simulink model "simulink_old_control_code"  (R2022b)
settings: Solver=FixedStepAuto  StartTime=0.0  StopTime=inf  FixedStep=0.0002  RelTol=1e-3
values from neighbouring files (symbols this model uses):
  bias_heave1 = 0    [setup_DAQ_simulink_temp.m]
  freq = 0.65    [setup_DAQ_simulink_temp.m]
  heave1 = hstar1*chord    [setup_DAQ_simulink_temp.m]
  phase = -60    [setup_DAQ_simulink_temp.m]
  phi = -90    [setup_DAQ_simulink_temp.m]
  srate = 1000    [setup_DAQ_simulink_temp.m]
  T = 1/srate    (= 0.001)    [setup_DAQ_simulink_temp.m]
undefined symbols (not defined in the file or in its folder): bias_forces, National_Instruments, PCIe, Wallace_cal_transpose
libraries: sldrtlib x13
settings Model: SimulationMode=external  ExtModeTrigPort=2  ExtModeTrigDuration=6000000  ExtModeTrigDurationFloating=inf  ExtModeTrigLevel=0.500000  Creator=xhe61  LastModifiedBy=ehandyca
settings DataIOCC: ReturnWorkspaceOutputs=off
settings HardwareCC: ProdBitPerLong=64  ProdHWDeviceType=Intel->x86-64 (Linux 64)
settings ModelReferenceCC: EnableRefExpFcnMdlSchedulingChecks=on
settings RTWCC: Description=Simulink Desktop Real-Time  SystemTargetFile=sldrt.tlc  TemplateMakefile=sldrt.tmf  RTWCompilerOptimization=on
settings CodeAppCC: MaxIdLength=95
settings SimulinkDesktopRealTimeCC: TargetLibSuffix=_sldrt.a  TargetPreCompLibLocation=C:\Program Files\MATLAB\R2022b\toolbox\sldrt\lib\win64

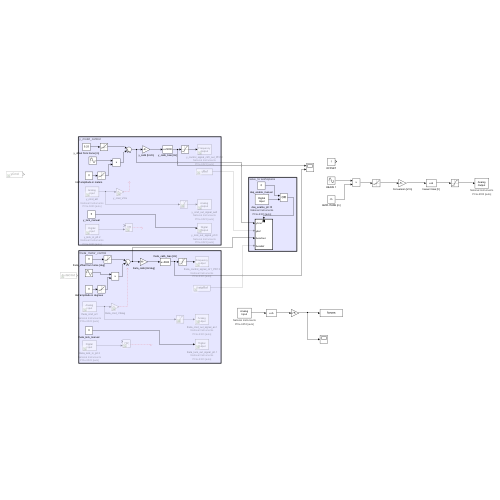
[thumbnail: Simulink's stored preview of the top-level diagram]
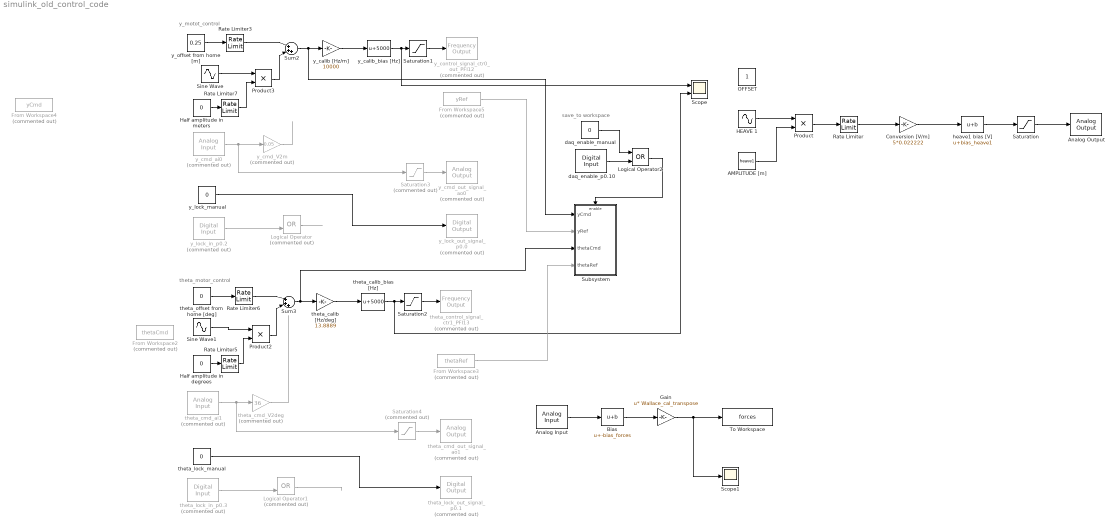
== system simulink_old_control_code ==
  note: save_to workspace
  note: theta_motor_control
  note: y_motot_control
  AMPLITUDE [m] : Constant  Value=heave1
  Analog Input : sldrtlib/Analog Input  SampleTime=T  MaxMissedTicks=10  ShowMissedTicks=off  YieldWhenWaiting=off  DrvName=National_Instruments/PCIe-6353  DrvAddress=4294967295  DrvOptions=[1 0 0 2 2 2 2]  Channels=[1:6]  RangeMode=1  VoltRange=1  DataType=1
      settings: AttributesFormatString=National Instruments\nPCIe-6353 [auto]
  Analog Output : sldrtlib/Analog Output  SampleTime=srate  MaxMissedTicks=10  ShowMissedTicks=off  YieldWhenWaiting=off  DrvName=National_Instruments/PCIe-6353  DrvAddress=4294967295  DrvOptions=[1 0 0 2 2 2 2]  Channels=1  RangeMode=1  VoltRange=1  InitialValue=[]  FinalValue=[]
      settings: AttributesFormatString=National Instruments\nPCIe-6353 [auto]
  Bias : Bias  Bias=-bias_forces  SaturateOnIntegerOverflow=off
  Conversion [V/m] : Gain  Gain=5*0.022222
  From Workspace2 : FromWorkspace  Commented=on  VariableName=thetaCmd  SampleTime=0.001  Interpolate=off  OutputAfterFinalValue=Cyclic repetition
  From Workspace3 : FromWorkspace  Commented=on  VariableName=thetaRef  SampleTime=0.001  Interpolate=off  OutputAfterFinalValue=Cyclic repetition
  From Workspace4 : FromWorkspace  Commented=on  VariableName=yCmd  SampleTime=0.001  Interpolate=off  OutputAfterFinalValue=Cyclic repetition
  From Workspace5 : FromWorkspace  Commented=on  VariableName=yRef  SampleTime=0.001  Interpolate=off  OutputAfterFinalValue=Cyclic repetition
  Gain : Gain  Gain=Wallace_cal_transpose  Multiplication=Matrix(u*K)
  HEAVE 1 : Sin  Frequency=freq  Phase=phase + phi  SampleTime=0
  Half amplitude in degrees : Constant  Value=0
  Half amplitude in meters : Constant  Value=0
  Logical Operator : Logic  Commented=on  Operator=OR  AllPortsSameDT=off  OutDataTypeStr=boolean
  Logical Operator1 : Logic  Commented=on  Operator=OR  AllPortsSameDT=off  OutDataTypeStr=boolean
  Logical Operator2 : Logic  Operator=OR  AllPortsSameDT=off  OutDataTypeStr=boolean
  OFFSET : Constant
  Product : Product
  Product2 : Product
  Product3 : Product
  Rate Limiter : RateLimiter  SampleTimeMode=inherited
  Rate Limiter3 : RateLimiter  RisingSlewLimit=0.04  FallingSlewLimit=-0.04  SampleTimeMode=inherited
  Rate Limiter5 : RateLimiter  RisingSlewLimit=10  FallingSlewLimit=-10  SampleTimeMode=inherited
  Rate Limiter6 : RateLimiter  RisingSlewLimit=15  FallingSlewLimit=-15  SampleTimeMode=inherited
  Rate Limiter7 : RateLimiter  RisingSlewLimit=0.01  FallingSlewLimit=-0.01  SampleTimeMode=inherited
  Saturation : Saturate  UpperLimit=10  LowerLimit=-10
  Saturation1 : Saturate  UpperLimit=10000  LowerLimit=5000
  Saturation2 : Saturate  UpperLimit=9200  LowerLimit=5000
  Saturation3 : Saturate  Commented=on  UpperLimit=10  LowerLimit=-10
  Saturation4 : Saturate  Commented=on  UpperLimit=10  LowerLimit=-10
  Scope : Scope  NumInputPorts=2
  Scope1 : Scope
  Sine Wave : Sin  Frequency=2*pi*0.65  SampleTime=0
  Sine Wave1 : Sin  Frequency=2*pi*0.65  Phase=-pi/2  SampleTime=0
  Subsystem : Subsystem
  Sum2 : Sum  Inputs=|+++
  Sum3 : Sum  Inputs=|+++
  To Workspace : ToWorkspace  VariableName=forces  SampleTime=-1
      settings: MaxDataPoints=20000  Save2DSignal=2-D array (concatenate along first dimension)
  daq_enable_manual : Constant  Value=0  OutDataTypeStr=boolean
  daq_enable_p0.10 : sldrtlib/Digital Input  SampleTime=0.001  MaxMissedTicks=10  ShowMissedTicks=off  YieldWhenWaiting=on  DrvName=National_Instruments/PCIe-6323  DrvAddress=4294967295  DrvOptions=[0 3 0 3 3 3 3]  Channels=11  BitMode=1  DataType=9
      settings: AttributesFormatString=National Instruments\nPCIe-6323 [auto]
  heave1 bias [V] : Bias  Bias=bias_heave1  SaturateOnIntegerOverflow=off
  theta_calib [Hz/deg] : Gain  Gain=13.8889
  theta_calib_bias [Hz] : Bias  Bias=5000  SaturateOnIntegerOverflow=off
  theta_cmd_V2deg : Gain  Commented=on  Gain=36
  theta_cmd_ai1 : sldrtlib/Analog Input  Commented=on  SampleTime=0.001  MaxMissedTicks=10  ShowMissedTicks=off  YieldWhenWaiting=off  DrvName=National_Instruments/PCIe-6323  DrvAddress=4294967295  DrvOptions=[0 3 61440 3 3 3 3]  Channels=2  RangeMode=1  VoltRange=1  DataType=1
      settings: AttributesFormatString=National Instruments\nPCIe-6323 [auto]
  theta_cmd_out_signal_ao1 : sldrtlib/Analog Output  Commented=on  SampleTime=0.001  MaxMissedTicks=10  ShowMissedTicks=off  YieldWhenWaiting=off  DrvName=National_Instruments/PCIe-6323  DrvAddress=4294967295  DrvOptions=[0 3 61440 3 3 3 3]  Channels=2  RangeMode=1  VoltRange=1  InitialValue=[]  FinalValue=[]
      settings: AttributesFormatString=National Instruments\nPCIe-6323 [auto]
  theta_control_signal_ctr1_PFI13 : sldrtlib/Frequency Output  Commented=on  SampleTime=T  MaxMissedTicks=10  ShowMissedTicks=off  YieldWhenWaiting=off  DrvName=National_Instruments/PCIe-6323  DrvAddress=4294967295  DrvOptions=[0 3 0 3 3 3 3]  Channels=2  FrequencySource=2  Frequency=[]  FrequencyFinalValue=[]  DutySource=1  Duty=0.5  DutyFinalValue=[]
      settings: AttributesFormatString=National Instruments\nPCIe-6323 [auto]
  theta_lock_in_p0.3 : sldrtlib/Digital Input  Commented=on  SampleTime=0.001  MaxMissedTicks=10  ShowMissedTicks=off  YieldWhenWaiting=on  DrvName=National_Instruments/PCIe-6323  DrvAddress=4294967295  DrvOptions=[0 3 61440 3 3 3 3]  Channels=4  BitMode=1  DataType=9
      settings: AttributesFormatString=National Instruments\nPCIe-6323 [auto]
  theta_lock_manual : Constant  Value=0  OutDataTypeStr=boolean
  theta_lock_out_signal_p0.1 : sldrtlib/Digital Output  Commented=on  SampleTime=T  MaxMissedTicks=10  ShowMissedTicks=off  YieldWhenWaiting=off  DrvName=National_Instruments/PCIe-6323  DrvAddress=4294967295  DrvOptions=[0 3 0 3 3 3 3]  Channels=2  BitMode=1  InitialValue=[]  FinalValue=[]
      settings: AttributesFormatString=National Instruments\nPCIe-6323 [auto]
  theta_offset from home [deg] : Constant  Value=0
  y_calib [Hz/m] : Gain  Gain=10000
  y_calib_bias [Hz] : Bias  Bias=5000  SaturateOnIntegerOverflow=off
  y_cmd_V2m : Gain  Commented=on  Gain=0.05
  y_cmd_ai0 : sldrtlib/Analog Input  Commented=on  SampleTime=0.001  MaxMissedTicks=10  ShowMissedTicks=off  YieldWhenWaiting=off  DrvName=National_Instruments/PCIe-6323  DrvAddress=4294967295  DrvOptions=[0 3 61440 3 3 3 3]  Channels=1  RangeMode=1  VoltRange=1  DataType=1
      settings: AttributesFormatString=National Instruments\nPCIe-6323 [auto]
  y_cmd_out_signal_ao0 : sldrtlib/Analog Output  Commented=on  SampleTime=0.001  MaxMissedTicks=10  ShowMissedTicks=off  YieldWhenWaiting=off  DrvName=National_Instruments/PCIe-6323  DrvAddress=4294967295  DrvOptions=[0 3 61440 3 3 3 3]  Channels=1  RangeMode=1  VoltRange=1  InitialValue=[]  FinalValue=[]
      settings: AttributesFormatString=National Instruments\nPCIe-6323 [auto]
  y_control_signal_ctr0_out_PFI12 : sldrtlib/Frequency Output  Commented=on  SampleTime=T  MaxMissedTicks=10  ShowMissedTicks=off  YieldWhenWaiting=off  DrvName=National_Instruments/PCIe-6323  DrvAddress=4294967295  DrvOptions=[0 3 0 3 3 3 3]  Channels=1  FrequencySource=2  Frequency=[]  FrequencyFinalValue=[]  DutySource=1  Duty=0.5  DutyFinalValue=[]
      settings: AttributesFormatString=National Instruments\nPCIe-6323 [auto]
  y_lock_in_p0.2 : sldrtlib/Digital Input  Commented=on  SampleTime=0.001  MaxMissedTicks=10  ShowMissedTicks=off  YieldWhenWaiting=on  DrvName=National_Instruments/PCIe-6323  DrvAddress=4294967295  DrvOptions=[0 3 61440 3 3 3 3]  Channels=3  BitMode=1  DataType=9
      settings: AttributesFormatString=National Instruments\nPCIe-6323 [auto]
  y_lock_manual : Constant  Value=0  OutDataTypeStr=boolean
  y_lock_out_signal_p0.0 : sldrtlib/Digital Output  Commented=on  SampleTime=T  MaxMissedTicks=10  ShowMissedTicks=off  YieldWhenWaiting=off  DrvName=National_Instruments/PCIe-6323  DrvAddress=4294967295  DrvOptions=[0 3 0 3 3 3 3]  Channels=1  BitMode=1  InitialValue=[]  FinalValue=[]
      settings: AttributesFormatString=National Instruments\nPCIe-6323 [auto]
  y_offset from home [m] : Constant  Value=0.25
  wires:
  y_lock_manual/1 -> y_lock_out_signal_p0.0/1
  theta_lock_in_p0.3/1 -> Logical Operator1/2
  theta_lock_manual/1 -> theta_lock_out_signal_p0.1/1
  y_cmd_ai0/1 -> Saturation3/1, y_cmd_V2m/1
  Logical Operator/1 -> ?
  Saturation4/1 -> theta_cmd_out_signal_ao1/1
  theta_cmd_ai1/1 -> theta_cmd_V2deg/1, Saturation4/1
  theta_cmd_V2deg/1 -> ?
  y_offset from home [m]/1 -> Rate Limiter3/1
  theta_calib [Hz/deg]/1 -> theta_calib_bias [Hz]/1
  Saturation2/1 -> theta_control_signal_ctr1_PFI13/1
  Sum3/1 -> Subsystem/3(thetaCmd), theta_calib [Hz/deg]/1
  theta_offset from home [deg]/1 -> Rate Limiter6/1
  Rate Limiter6/1 -> Sum3/1
  Logical Operator1/1 -> ?
  Sum2/1 -> Subsystem/1(yCmd), y_calib [Hz/m]/1
  Saturation3/1 -> y_cmd_out_signal_ao0/1
  y_lock_in_p0.2/1 -> Logical Operator/2
  Saturation1/1 -> y_control_signal_ctr0_out_PFI12/1
  theta_calib_bias [Hz]/1 -> Scope/2, Saturation2/1
  y_calib [Hz/m]/1 -> y_calib_bias [Hz]/1
  Rate Limiter3/1 -> Sum2/1
  y_calib_bias [Hz]/1 -> Scope/1, Saturation1/1
  y_cmd_V2m/1 -> ?
  Logical Operator2/1 -> Subsystem/Enable
  daq_enable_p0.10/1 -> Logical Operator2/2
  daq_enable_manual/1 -> Logical Operator2/1
  Sine Wave1/1 -> Product2/1
  Half amplitude in degrees/1 -> Rate Limiter5/1
  Rate Limiter5/1 -> Product2/2
  Product2/1 -> Sum3/2
  From Workspace3/1 -> Subsystem/4(thetaRef)
  Half amplitude in meters/1 -> Rate Limiter7/1
  Sine Wave/1 -> Product3/1
  Product3/1 -> Sum2/2
  Rate Limiter7/1 -> Product3/2
  From Workspace5/1 -> Subsystem/2(yRef)
  Analog Input/1 -> Bias/1
  Gain/1 -> Scope1/1, To Workspace/1
  Bias/1 -> Gain/1
  Conversion [V/m]/1 -> heave1 bias [V]/1
  heave1 bias [V]/1 -> Saturation/1
  Saturation/1 -> Analog Output/1
  Rate Limiter/1 -> Conversion [V/m]/1
  HEAVE 1/1 -> Product/1
  Product/1 -> Rate Limiter/1
  AMPLITUDE [m]/1 -> Product/2

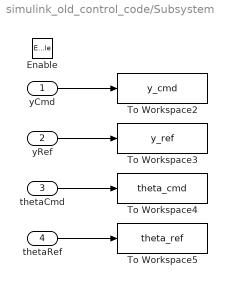
== system simulink_old_control_code/Subsystem ==
  yCmd : Inport
  yRef : Inport  Port=2
  thetaCmd : Inport  Port=3
  thetaRef : Inport  Port=4
  Enable : EnablePort
  To Workspace2 : ToWorkspace  VariableName=y_cmd  SampleTime=0.001
      settings: Save2DSignal=2-D array (concatenate along first dimension)
  To Workspace3 : ToWorkspace  VariableName=y_ref  SampleTime=0.001
      settings: Save2DSignal=2-D array (concatenate along first dimension)
  To Workspace4 : ToWorkspace  VariableName=theta_cmd  SampleTime=0.001
      settings: Save2DSignal=2-D array (concatenate along first dimension)
  To Workspace5 : ToWorkspace  VariableName=theta_ref  SampleTime=0.001
      settings: Save2DSignal=2-D array (concatenate along first dimension)
  wires:
  yRef/1 -> To Workspace3/1
  yCmd/1 -> To Workspace2/1
  thetaCmd/1 -> To Workspace4/1
  thetaRef/1 -> To Workspace5/1
